simulink model "full_r2016b"  (R2019b)
settings: Solver=VariableStepAuto  StartTime=0.0  StopTime=10.0  RelTol=1e-3
libraries: aerolibgravity2 x2, aerolibconvert2 x1, vrlib x1
settings Model: Creator=decla  LastModifiedBy=decla
settings DebuggingCC: ArithmeticOperatorsInVariantConditions=warning
settings SFSimCC: CustomCodeUndefinedFunction=UseInterfaceOnly
settings CodeAppCC: StateflowObjectComments=on

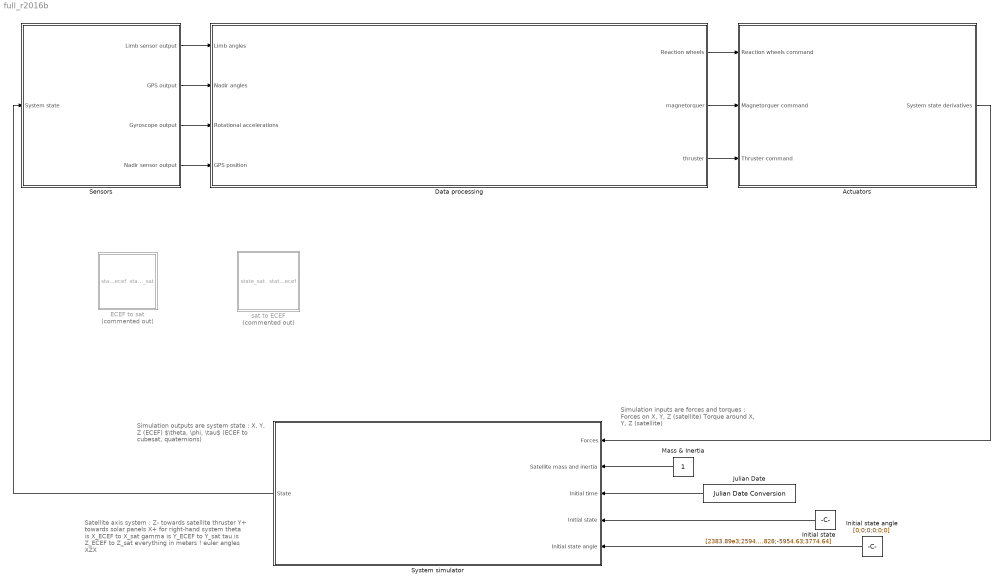
== system full_r2016b ==
  note: Simulation outputs are system state :
      | X, Y, Z (ECEF)
      | $\theta, \phi, \tau$ (ECEF to cubesat, quaternions)
  note: Simulation inputs are forces and torques :
      | Forces on X, Y, Z (satellite)
      | Torque around X, Y, Z (satellite)
  note: Satellite axis system :
      | Z- towards satellite thruster
      | Y+ towards solar panels
      | X+ for right-hand system
      | theta is X_ECEF to X_sat
      | gamma is Y_ECEF to Y_sat
      | tau is Z_ECEF to Z_sat
      | everything in meters !
      | euler angles XZX
  Actuators : Subsystem
  Data processing : Subsystem
  ECEF to sat : MATLAB Function  Commented=on  TreatAsAtomicUnit=on
  Initial state : Constant  Value=[2383.89e3;2594.67e3;5906.12e3;-2871.828;-5954.63;3774.64]
  Initial state angle : Constant  Value=[0;0;0;0;0;0]
  Julian Date : aerolibconvert2/Julian Date Conversion  year=2004  month=October  day=10  hour=12  min=21  sec=0  modflag=off  deltaT=None  errorflag=Error
      settings: SourceProductBaseCode=AE
  Mass & Inertia : Constant
  Sensors : Subsystem
  System simulator : Subsystem
  sat to ECEF : MATLAB Function  Commented=on  TreatAsAtomicUnit=on
  wires:
  Data processing/3(thruster) -> Actuators/3(Thruster command)
  Actuators/1(System state derivatives) -> System simulator/1(Forces)
  System simulator/1(State) -> Sensors/1(System state)
  Sensors/4(Nadir sensor output) -> Data processing/4(GPS position)
  Sensors/3(Gyroscope output) -> Data processing/3(Rotational accelerations)
  Sensors/2(GPS output) -> Data processing/2(Nadir angles)
  Sensors/1(Limb sensor output) -> Data processing/1(Limb angles)
  Data processing/2(magnetorquer) -> Actuators/2(Magnetorquer command)
  Data processing/1(Reaction wheels) -> Actuators/1(Reaction wheels command)
  Mass & Inertia/1 -> System simulator/2(Satellite mass and inertia)
  Julian Date/1 -> System simulator/3(Initial time)
  Initial state/1 -> System simulator/4(Initial state)
  Initial state angle/1 -> System simulator/5(Initial state angle)

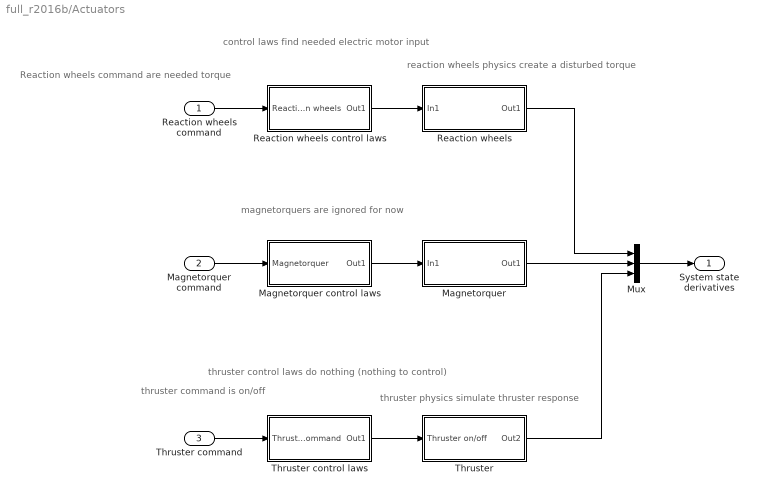
== system full_r2016b/Actuators ==
  note: magnetorquers are ignored for now
  note: thruster control laws do nothing (nothing to control)
  note: thruster physics simulate thruster response
  note: thruster command is on/off
  note: reaction wheels physics create a disturbed torque
  note: control laws find needed electric motor input
  note: Reaction wheels command are needed torque
  Reaction wheels command : Inport
  Magnetorquer command : Inport  Port=2
  Thruster command : Inport  Port=3
  Magnetorquer : Subsystem
  Magnetorquer control laws : Subsystem
  Mux : Mux  Inputs=3
  Reaction wheels : Subsystem
  Reaction wheels control laws : Subsystem
  Thruster : Subsystem
  Thruster control laws : Subsystem
  System state derivatives : Outport
  wires:
  Reaction wheels command/1 -> Reaction wheels control laws/1(Reaction wheels)
  Magnetorquer command/1 -> Magnetorquer control laws/1(Magnetorquer)
  Thruster command/1 -> Thruster control laws/1(Thruster command)
  Thruster control laws/1(Out1) -> Thruster/1(Thruster on/off)
  Magnetorquer control laws/1(Out1) -> Magnetorquer/1(In1)
  Reaction wheels control laws/1(Out1) -> Reaction wheels/1(In1)
  Thruster/1(Out2) -> Mux/3
  Magnetorquer/1(Out1) -> Mux/2
  Reaction wheels/1(Out1) -> Mux/1
  Mux/1 -> System state derivatives/1

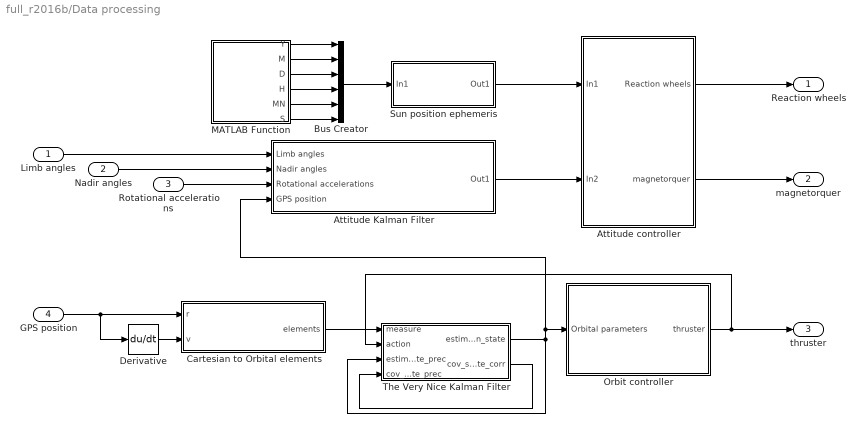
== system full_r2016b/Data processing ==
  Limb angles : Inport
  Nadir angles : Inport  Port=2
  Rotational accelerations : Inport  Port=3
  GPS position : Inport  Port=4
  Attitude Kalman Filter : Subsystem
  Attitude controller : Subsystem
  Bus Creator : BusCreator  Inputs=6
  Cartesian to Orbital elements : MATLAB Function  TreatAsAtomicUnit=on
  Derivative : Derivative
  MATLAB Function : MATLAB Function  TreatAsAtomicUnit=on
  Orbit controller : Subsystem
  Sun position ephemeris : Subsystem
  The Very Nice Kalman Filter : MATLAB Function  TreatAsAtomicUnit=on
  Reaction wheels : Outport
  magnetorquer : Outport  Port=2
  thruster : Outport  Port=3
  wires:
  Limb angles/1 -> Attitude Kalman Filter/1(Limb angles)
  Nadir angles/1 -> Attitude Kalman Filter/2(Nadir angles)
  Rotational accelerations/1 -> Attitude Kalman Filter/3(Rotational accelerations)
  Orbit controller/1(thruster) -> The Very Nice Kalman Filter/2(action), thruster/1
  Attitude controller/1(Reaction wheels) -> Reaction wheels/1
  Attitude controller/2(magnetorquer) -> magnetorquer/1
  MATLAB Function/1(Y) -> Bus Creator/1
  MATLAB Function/2(M) -> Bus Creator/2
  MATLAB Function/3(D) -> Bus Creator/3
  MATLAB Function/4(H) -> Bus Creator/4
  MATLAB Function/5(MN) -> Bus Creator/5
  MATLAB Function/6(S) -> Bus Creator/6
  Bus Creator/1 -> Sun position ephemeris/1(In1)
  Sun position ephemeris/1(Out1) -> Attitude controller/1(In1)
  Attitude Kalman Filter/1(Out1) -> Attitude controller/2(In2)
  Cartesian to Orbital elements/1(elements) -> The Very Nice Kalman Filter/1(measure)
  Derivative/1 -> Cartesian to Orbital elements/2(v)
  GPS position/1 -> Cartesian to Orbital elements/1(r), Derivative/1
  The Very Nice Kalman Filter/1(estimation_state) -> The Very Nice Kalman Filter/3(estimation_state_prec), Attitude Kalman Filter/4(GPS position), Orbit controller/1(Orbital parameters)
  The Very Nice Kalman Filter/2(cov_state_corr) -> The Very Nice Kalman Filter/4(cov_state_prec)

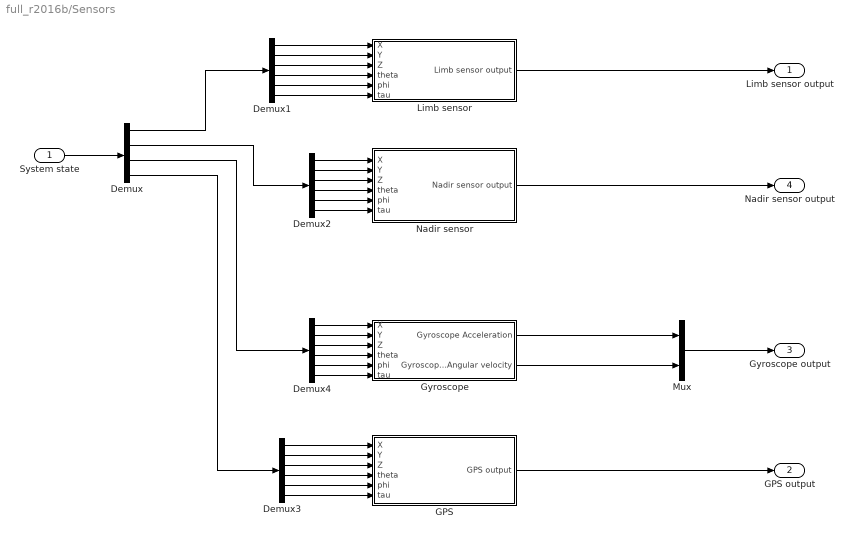
== system full_r2016b/Sensors ==
  System state : Inport
  Demux : Demux
  Demux{1..4} (4 alike) : Demux  Outputs=6
  GPS : Subsystem
  Gyroscope : Subsystem
  Limb sensor : Subsystem
  Mux : Mux  Inputs=2
  Nadir sensor : Subsystem
  Limb sensor output : Outport
  GPS output : Outport  Port=2
  Gyroscope output : Outport  Port=3
  Nadir sensor output : Outport  Port=4
  wires:
  Mux/1 -> Gyroscope output/1
  Demux1/1 -> Limb sensor/1(X)
  Demux1/4 -> Limb sensor/4(theta)
  Demux4/2 -> Gyroscope/2(Y)
  Demux1/5 -> Limb sensor/5(phi)
  Demux1/2 -> Limb sensor/2(Y)
  Demux3/1 -> GPS/1(X)
  Demux2/3 -> Nadir sensor/3(Z)
  Demux1/3 -> Limb sensor/3(Z)
  Demux4/1 -> Gyroscope/1(X)
  Demux3/3 -> GPS/3(Z)
  Demux2/6 -> Nadir sensor/6(tau)
  Limb sensor/1("Limb sensor output ") -> Limb sensor output/1
  GPS/1(GPS output) -> GPS output/1
  Demux4/3 -> Gyroscope/3(Z)
  Demux1/6 -> Limb sensor/6(tau)
  Demux3/4 -> GPS/4(theta)
  Demux2/1 -> Nadir sensor/1(X)
  Demux2/5 -> Nadir sensor/5(phi)
  Demux/1 -> Demux1/1
  Demux3/6 -> GPS/6(tau)
  Demux2/4 -> Nadir sensor/4(theta)
  Demux/3 -> Demux4/1
  Gyroscope/1(Gyroscope Acceleration) -> Mux/1
  Demux2/2 -> Nadir sensor/2(Y)
  Nadir sensor/1(Nadir sensor output) -> Nadir sensor output/1
  Gyroscope/2(Gyroscope Angular velocity) -> Mux/2
  Demux/4 -> Demux3/1
  Demux4/5 -> Gyroscope/5(phi)
  Demux4/4 -> Gyroscope/4(theta)
  Demux3/2 -> GPS/2(Y)
  Demux/2 -> Demux2/1
  Demux3/5 -> GPS/5(phi)
  Demux4/6 -> Gyroscope/6(tau)
  System state/1 -> Demux/1

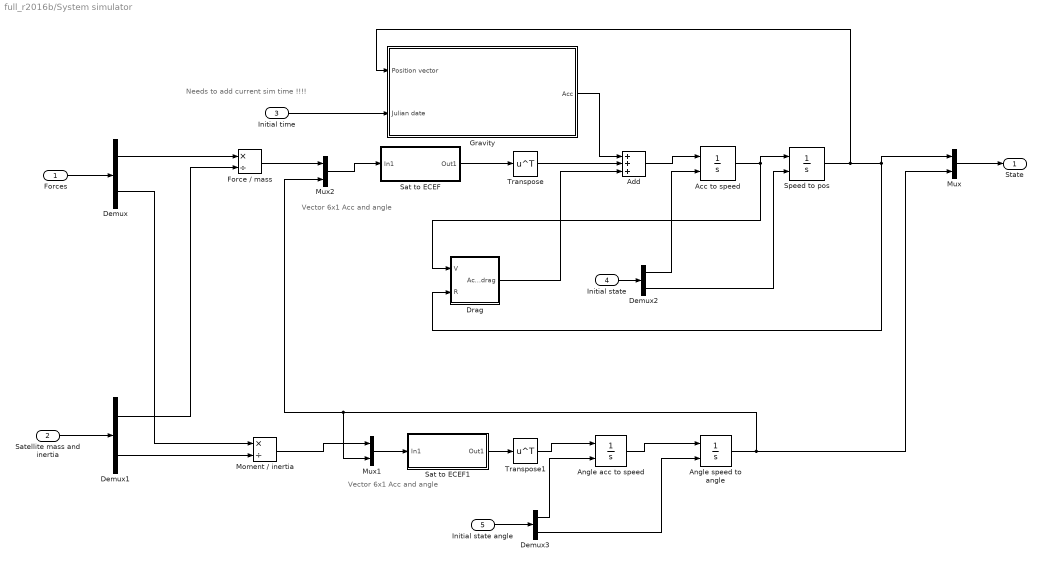
== system full_r2016b/System simulator ==
  note: Vector 6x1
      | Acc and angle
  note: Vector 6x1
      | Acc and angle
  note: Needs to add current sim time !!!!
  Forces : Inport
  Satellite mass and inertia : Inport  Port=2
  Initial time : Inport  Port=3
  Initial state : Inport  Port=4
  Initial state angle : Inport  Port=5
  Acc to speed : Integrator  InitialConditionSource=external  InitialCondition=[-2871.828;-5954.63;3774.64]
  Add : Sum  Inputs=+++
  Angle acc to speed : Integrator  InitialConditionSource=external
  Angle speed to angle : Integrator  InitialConditionSource=external
  Demux{,1..3} (4 alike) : Demux  Outputs=2
  Drag : Subsystem
  Force / mass : Product  Inputs=*/
  Gravity : Subsystem
  Moment / inertia : Product  Inputs=*/
  Mux : Mux  Inputs=2
  Mux1 : Mux  Inputs=2
  Mux2 : Mux  Inputs=2
  Sat to ECEF : Subsystem
  Sat to ECEF1 : Subsystem
  Speed to pos : Integrator  InitialConditionSource=external  InitialCondition=[2383.89e3;2594.67e3;5906.12e3]
  Transpose : Math  Operator=transpose  SaturateOnIntegerOverflow=on
  Transpose1 : Math  Operator=transpose  SaturateOnIntegerOverflow=on
  State : Outport
  wires:
  Add/1 -> Acc to speed/1
  Moment / inertia/1 -> Mux1/1
  Mux1/1 -> Sat to ECEF1/1(In1)
  Forces/1 -> Demux/1
  Force / mass/1 -> Mux2/1
  Mux2/1 -> Sat to ECEF/1(In1)
  Demux/1 -> Force / mass/1
  Demux1/2 -> Moment / inertia/2
  Mux/1 -> State/1
  Satellite mass and inertia/1 -> Demux1/1
  Angle speed to angle/1 -> Mux1/2, Mux2/2, Mux/2
  Sat to ECEF1/1(Out1) -> Transpose1/1
  Demux3/1 -> Angle acc to speed/2
  Initial state angle/1 -> Demux3/1
  Transpose/1 -> Add/2
  Demux3/2 -> Angle speed to angle/2
  Demux/2 -> Moment / inertia/1
  Transpose1/1 -> Angle acc to speed/1
  Demux2/2 -> Speed to pos/2
  Speed to pos/1 -> Mux/1, Drag/2(R), Gravity/1(Position vector)
  Gravity/1(Acc) -> Add/1
  Initial time/1 -> Gravity/2(Julian date)
  Angle acc to speed/1 -> Angle speed to angle/1
  Demux1/1 -> Force / mass/2
  Initial state/1 -> Demux2/1
  Acc to speed/1 -> Drag/1(V), Speed to pos/1
  Drag/1(Acc_drag) -> Add/3
  Demux2/1 -> Acc to speed/2
  Sat to ECEF/1(Out1) -> Transpose/1

== system full_r2016b/Actuators/Magnetorquer ==
  In1 : Inport
  Out1 : Outport
  wires:
  In1/1 -> Out1/1

== system full_r2016b/Actuators/Magnetorquer control laws ==
  Magnetorquer : Inport
  Out1 : Outport
  wires:
  Magnetorquer/1 -> Out1/1

== system full_r2016b/Actuators/Reaction wheels ==
  In1 : Inport
  Out1 : Outport
  wires:
  In1/1 -> Out1/1

== system full_r2016b/Actuators/Reaction wheels control laws ==
  Reaction wheels : Inport
  X wheel inertia : Constant
  Y wheel inertia1 : Constant
  Z wheel inertia1 : Constant
  Out1 : Outport
  wires:
  Reaction wheels/1 -> Out1/1

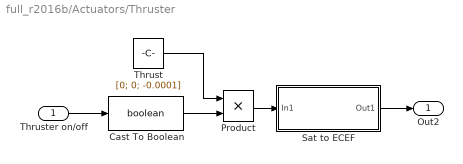
== system full_r2016b/Actuators/Thruster ==
  Thruster on/off : Inport
  Cast To Boolean : DataTypeConversion  OutDataTypeStr=boolean
  Product : Product
  Sat to ECEF : Subsystem
  Thrust : Constant  Value=[0; 0; -0.0001]
  Out2 : Outport
  wires:
  Product/1 -> Sat to ECEF/1(In1)
  Thrust/1 -> Product/1
  Thruster on/off/1 -> Cast To Boolean/1
  Sat to ECEF/1(Out1) -> Out2/1
  Cast To Boolean/1 -> Product/2

== system full_r2016b/Actuators/Thruster control laws ==
  Thruster command : Inport
  Out1 : Outport
  wires:
  Thruster command/1 -> Out1/1

== system full_r2016b/Data processing/Attitude Kalman Filter ==
  Limb angles : Inport
  Nadir angles : Inport  Port=2
  Rotational accelerations : Inport  Port=3
  GPS position : Inport  Port=4
  Out1 : Outport
  wires:
  Limb angles/1 -> Out1/1

== system full_r2016b/Data processing/Attitude controller ==
  In1 : Inport
  In2 : Inport  Port=2
  Command : Subsystem
  Control : Subsystem
  Reaction wheels : Outport
  magnetorquer : Outport  Port=2
  wires:
  In2/1 -> Control/3(In3)
  In1/1 -> Control/2(In2)
  Control/2(magnetorquer) -> magnetorquer/1
  Control/1(Reaction wheels) -> Reaction wheels/1
  Command/1(Out1) -> Control/1(In1)

== system full_r2016b/Data processing/Orbit controller ==
  Orbital parameters : Inport
  Command : Subsystem
  Control : Subsystem
  thruster : Outport
  wires:
  Command/1(Out1) -> Control/2(In1)
  Orbital parameters/1 -> Control/1(Orbital parameters)
  Control/1(Out1) -> thruster/1

== system full_r2016b/Data processing/Sun position ephemeris ==
  In1 : Inport
  Out1 : Outport
  wires:
  In1/1 -> Out1/1

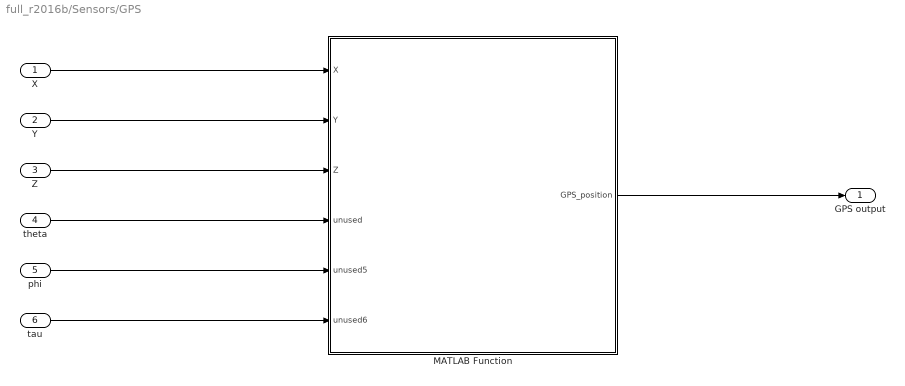
== system full_r2016b/Sensors/GPS ==
  X : Inport
  Y : Inport  Port=2
  Z : Inport  Port=3
  theta : Inport  Port=4
  phi : Inport  Port=5
  tau : Inport  Port=6
  MATLAB Function : MATLAB Function  TreatAsAtomicUnit=on
  GPS output : Outport
  wires:
  MATLAB Function/1(GPS_position) -> GPS output/1
  X/1 -> MATLAB Function/1(X)
  Y/1 -> MATLAB Function/2(Y)
  Z/1 -> MATLAB Function/3(Z)
  theta/1 -> MATLAB Function/4(unused)
  phi/1 -> MATLAB Function/5(unused5)
  tau/1 -> MATLAB Function/6(unused6)

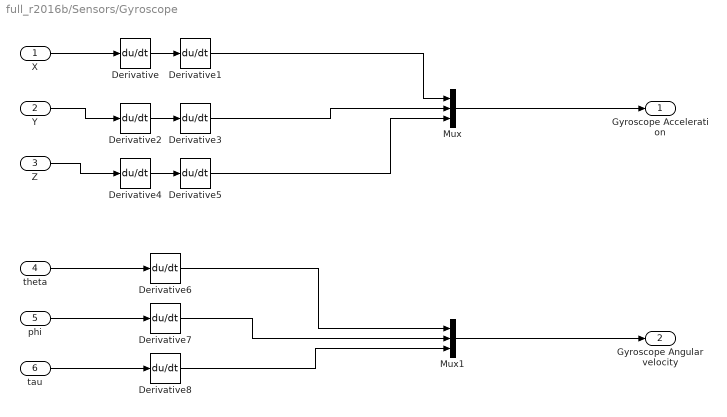
== system full_r2016b/Sensors/Gyroscope ==
  X : Inport
  Y : Inport  Port=2
  Z : Inport  Port=3
  theta : Inport  Port=4
  phi : Inport  Port=5
  tau : Inport  Port=6
  Derivative{,1..8} (9 alike) : Derivative
  Mux : Mux  Inputs=3
  Mux1 : Mux  Inputs=3
  Gyroscope Acceleration : Outport
  Gyroscope Angular velocity : Outport  Port=2
  wires:
  Derivative/1 -> Derivative1/1
  Derivative1/1 -> Mux/1
  X/1 -> Derivative/1
  Derivative2/1 -> Derivative3/1
  Derivative3/1 -> Mux/2
  Derivative4/1 -> Derivative5/1
  Derivative5/1 -> Mux/3
  Mux/1 -> Gyroscope Acceleration/1
  Z/1 -> Derivative4/1
  Y/1 -> Derivative2/1
  theta/1 -> Derivative6/1
  phi/1 -> Derivative7/1
  tau/1 -> Derivative8/1
  Derivative6/1 -> Mux1/1
  Derivative7/1 -> Mux1/2
  Derivative8/1 -> Mux1/3
  Mux1/1 -> Gyroscope Angular velocity/1

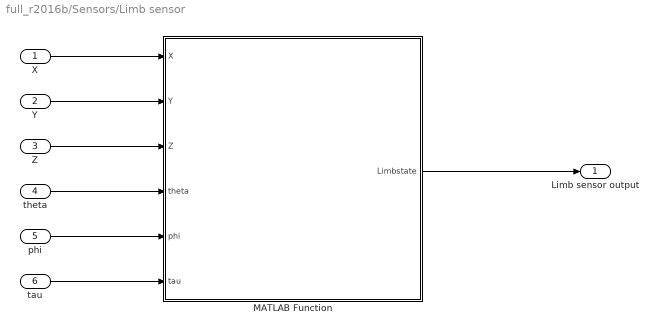
== system full_r2016b/Sensors/Limb sensor ==
  X : Inport
  Y : Inport  Port=2
  Z : Inport  Port=3
  theta : Inport  Port=4
  phi : Inport  Port=5
  tau : Inport  Port=6
  MATLAB Function : MATLAB Function  TreatAsAtomicUnit=on
  "Limb sensor output " : Outport
  wires:
  X/1 -> MATLAB Function/1(X)
  MATLAB Function/1(Limbstate) -> "Limb sensor output "/1
  tau/1 -> MATLAB Function/6(tau)
  phi/1 -> MATLAB Function/5(phi)
  theta/1 -> MATLAB Function/4(theta)
  Z/1 -> MATLAB Function/3(Z)
  Y/1 -> MATLAB Function/2(Y)

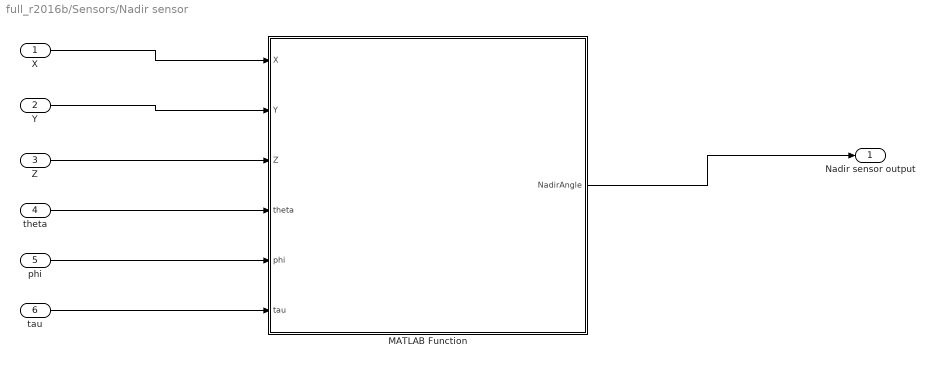
== system full_r2016b/Sensors/Nadir sensor ==
  X : Inport
  Y : Inport  Port=2
  Z : Inport  Port=3
  theta : Inport  Port=4
  phi : Inport  Port=5
  tau : Inport  Port=6
  MATLAB Function : MATLAB Function  TreatAsAtomicUnit=on
  Nadir sensor output : Outport
  wires:
  MATLAB Function/1(NadirAngle) -> Nadir sensor output/1
  X/1 -> MATLAB Function/1(X)
  Y/1 -> MATLAB Function/2(Y)
  Z/1 -> MATLAB Function/3(Z)
  theta/1 -> MATLAB Function/4(theta)
  phi/1 -> MATLAB Function/5(phi)
  tau/1 -> MATLAB Function/6(tau)

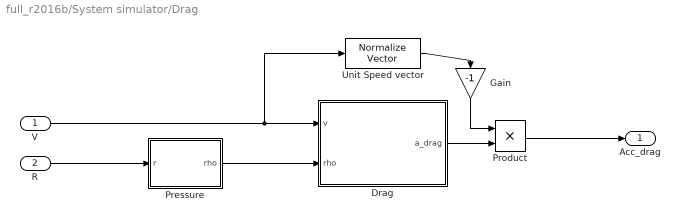
== system full_r2016b/System simulator/Drag ==
  V : Inport
  R : Inport  Port=2
  Drag : MATLAB Function  TreatAsAtomicUnit=on
  Gain : Gain  Gain=-1
  Pressure : MATLAB Function  TreatAsAtomicUnit=on
  Product : Product
  Unit Speed vector : vrlib/Utilities/Normalize Vector  maxzero=0
  Acc_drag : Outport
  wires:
  Pressure/1(rho) -> Drag/2(rho)
  V/1 -> Unit Speed vector/1, Drag/1(v)
  R/1 -> Pressure/1(r)
  Unit Speed vector/1 -> Gain/1
  Product/1 -> Acc_drag/1
  Drag/1(a_drag) -> Product/2
  Gain/1 -> Product/1

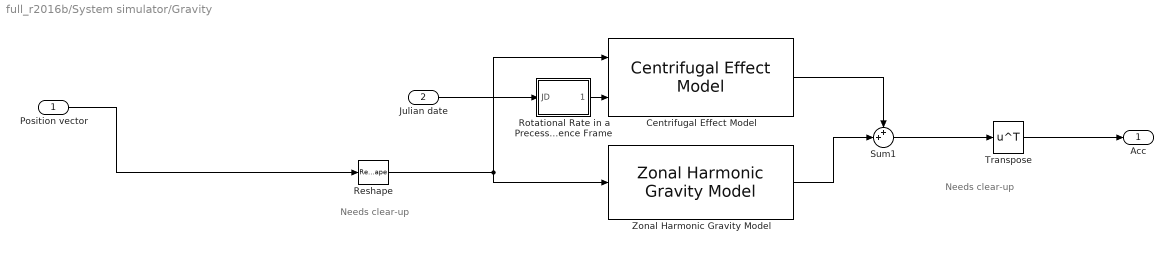
== system full_r2016b/System simulator/Gravity ==
  note: Needs clear-up
  note: Needs clear-up
  Position vector : Inport
  Julian date : Inport  Port=2
  Centrifugal Effect Model : aerolibgravity2/Centrifugal Effect Model  ptype=Custom  omega=7.2921150e-005  rate_loc=on
      settings: SourceProductBaseCode=AE
  Reshape : Reshape  OutputDimensionality=Row vector (2-D)
  Rotational Rate in a Precessing Reference Frame : Subsystem
  Sum1 : Sum  Inputs=++|
  Transpose : Math  Operator=transpose  SignedPower=on  SaturateOnIntegerOverflow=on
  Zonal Harmonic Gravity Model : aerolibgravity2/Zonal Harmonic Gravity Model  units=Metric (MKS)  degree=4  action=Warning  ptype=Earth  R=6378136.3  GM=398600441500000  jvalue=[1.0826269e-03 -2.5323000e-06 -1.6204000e-06]
      settings: SourceProductBaseCode=AE
  Acc : Outport
  wires:
  Reshape/1 -> Centrifugal Effect Model/1, Zonal Harmonic Gravity Model/1
  Rotational Rate in a Precessing Reference Frame/1(omega) -> Centrifugal Effect Model/2
  Position vector/1 -> Reshape/1
  Julian date/1 -> Rotational Rate in a Precessing Reference Frame/1(JD)
  Zonal Harmonic Gravity Model/1 -> Sum1/2
  Centrifugal Effect Model/1 -> Sum1/1
  Sum1/1 -> Transpose/1
  Transpose/1 -> Acc/1

== system full_r2016b/System simulator/Sat to ECEF ==
  In1 : Inport
  SAT TO ECEF : MATLAB Function  TreatAsAtomicUnit=on
  Out1 : Outport
  wires:
  In1/1 -> SAT TO ECEF/1(state_sat)
  SAT TO ECEF/1(state_ecef) -> Out1/1

== system full_r2016b/System simulator/Sat to ECEF1 ==
  In1 : Inport
  SAT TO ECEF : MATLAB Function  TreatAsAtomicUnit=on
  Out1 : Outport
  wires:
  In1/1 -> SAT TO ECEF/1(state_sat)
  SAT TO ECEF/1(state_ecef) -> Out1/1

== system full_r2016b/Actuators/Thruster/Sat to ECEF ==
  In1 : Inport
  Out1 : Outport
  wires:
  In1/1 -> Out1/1

== system full_r2016b/Data processing/Attitude controller/Command ==
  In1 : Inport
  Out1 : Outport
  wires:
  In1/1 -> Out1/1

== system full_r2016b/Data processing/Attitude controller/Control ==
  In1 : Inport
  In2 : Inport  Port=2
  In3 : Inport  Port=3
  Reaction wheels : Outport
  magnetorquer : Outport  Port=2
  wires:
  In1/1 -> Reaction wheels/1

== system full_r2016b/Data processing/Orbit controller/Command ==
  In1 : Inport
  Constant : Constant
  Out1 : Outport
  wires:
  In1/1 -> Out1/1

== system full_r2016b/Data processing/Orbit controller/Control ==
  Orbital parameters : Inport
  In1 : Inport  Port=2
  Out1 : Outport
  wires:
  Orbital parameters/1 -> Out1/1

== system full_r2016b/System simulator/Gravity/Rotational Rate in a Precessing Reference Frame ==
  JD : Inport
  Bias : Bias  Bias=-2451545
  Bias1 : Bias  Bias=7.086e-12
  Bias2 : Bias  Bias=7.2921151467e-5
  Gain : Gain  Gain=4.3e-15/36525
  omega : Outport
  wires:
  JD/1 -> Bias/1
  Bias/1 -> Gain/1
  Gain/1 -> Bias1/1
  Bias1/1 -> Bias2/1
  Bias2/1 -> omega/1

== matlab function full_r2016b/ECEF to sat ==
  data: state_ecef input; state_sat output
function state_sat = fcn(state_ecef)

    x = state(0)
    y = state(1)
    z = state(2)
    theta = state(3)
    phi = state(4)
    tau = state(5)

    % from https://en.wikipedia.org/wiki/Euler_angles
    c1 = cos(theta)
    c2 = cos(phi)
    c3 = cos(tau)
    s1 = sin(theta)
    s2 = sin(phi)
    s3 = sin(tau)
    XZX = [
       c2, -c3*c2, s2*s3;
       c1*s2, c1*c2*c3-s1*s3, -c3*s1-c1*c2*s3;
       s1*s2, c1*s3+c2*c3*s1, c1*c3-c2*s1*s3
    ];
    
    state_sat =[x;y;z]*XZX;

== matlab function full_r2016b/Data processing/MATLAB Function ==
  data: Y output; M output; D output; H output; MN output; S output
% https://www.mathworks.com/matlabcentral/answers/30479-how-to-get-system-date-and-time-into-simulink
function [Y, M, D, H, MN, S] = sysClock()
   coder.extrinsic('clock');
   Y = 0;
   M = 0;
   D = 0;
   H = 0;
   MN = 0;
   S = 0;
   [Y, M, D, H, MN, S] = clock;
end

== matlab function full_r2016b/System simulator/Drag/Drag ==
  data: v input; a_drag output; rho input
function a_drag = fcn(v, rho)
area = 100e-4;
mass = 3;
V = norm(v);
Cd = 1.05;

a_drag = -0.5*Cd*(area/mass)*rho*V^2;

== matlab function full_r2016b/System simulator/Drag/Pressure ==
  data: r input; rho output
function rho = fcn(r)
alt = norm(r);
A = 1.140564e-10;
B = -2.130756e-7;
C = 1.570562e-4;
D = -0.07029296;
E = -12.89844;

rho = exp(A*alt^4 + B*alt^3 + C*alt^2 + D*alt + E);

== matlab function full_r2016b/Sensors/GPS/MATLAB Function ==
  data: X input; GPS_position output; Y input; Z input; unused input; unused5 input; unused6 input
function GPS_position    = GPS_function(X, Y, Z, ~, ~, ~)


noise_pos = 0 + (10-0) .* rand(1,1); % bruit pour la position X
GPS_position_x = X + noise_pos;
noise_pos = 0 + (10-0) .* rand(1,1); % bruit pour la position Y
GPS_position_y = Y + noise_pos;
noise_pos = 0 + (10-0) .* rand(1,1); % bruit pour la position Z
GPS_position_z = Z + noise_pos;

GPS_position = [GPS_position_x; GPS_position_y; GPS_position_z];
end

== matlab function full_r2016b/Sensors/Limb sensor/MATLAB Function ==
  data: X input; Limbstate output; Y input; Z input; theta input; phi input; tau input
function Limbstate  = Limb_function(X, Y, Z, theta, phi, tau)
% Take as input the postition X,Y,Z and the attitude Theta (rotX), phi
% (rotY), tau (rotZ).
% Return the limb state in ECEF ref 

noise = 0 + (0.25-0) .* rand(1,1);
LimbAngle = acrtan(6371000/ sqrt(X^2 + Y^2 + Z^2)) + noise; % Tan(angle) = opposite * Adj

tau2limb = tau - limbAngle  % angle between tau and limb  




c1 = cos(theta)
c2 = cos(phi)
c3 = cos(tau2limb)
s1 = sin(theta)
s2 = sin(phi)
s3 = sin(tau2limb)
XZX = [
c2, -c3*c2, s2*s3;
c1*s2, c1*c2*c3-s1*s3, -c3*s1-c1*c2*s3;
s1*s2, c1*s3+c2*c3*s1, c1*c3-c2*s1*s3
];

Limbstate =[X;Y;Z]*(XZX');

end

== matlab function full_r2016b/Sensors/Nadir sensor/MATLAB Function ==
  data: X input; NadirAngle output; Y input; Z input; theta input; phi input; tau input
function NadirAngle   = Nadir_function(X, Y, Z, theta, phi, tau)
% En faisant l'hypothèse que SystemStates = ([rotX rotY rotZ],[X Y Z])
noise = 0 + (0.25-0) .* rand(1,1);
NadirAngle_x = -X + noise;
noise = 0 + (0.25-0) .* rand(1,1);
NadirAngle_y = -Y + noise;
noise = 0 + (0.25-0) .* rand(1,1);
NadirAngle_z = -Z + noise;


vector = -1 .* [NadirAngle_x, NadirAngle_y, NadirAngle_z];

unit_vector = vector / (sqrt(NadirAngle_x^2 + NadirAngle_y^2 + NadirAngle_z^2)


% from https://en.wikipedia.org/wiki/Euler_angles
c1 = cos(theta)
c2 = cos(phi)
c3 = cos(tau)
s1 = sin(theta)
s2 = sin(phi)
s3 = sin(tau)
XZX = [
c2, -c3*c2, s2*s3;
c1*s2, c1*c2*c3-s1*s3, -c3*s1-c1*c2*s3;
s1*s2, c1*s3+c2*c3*s1, c1*c3-c2*s1*s3
];

state_sat =unit_vector .* XZX;
end

== matlab function full_r2016b/sat to ECEF ==
  data: state_sat input; state_ecef output
function state_ecef = fcn(state_sat)

    x = state(0)
    y = state(1)
    z = state(2)
    theta = state(3)
    phi = state(4)
    tau = state(5)

    % from https://en.wikipedia.org/wiki/Euler_angles
    c1 = cos(theta)
    c2 = cos(phi)
    c3 = cos(tau)
    s1 = sin(theta)
    s2 = sin(phi)
    s3 = sin(tau)
    XZX = [
       c2, -c3*c2, s2*s3;
       c1*s2, c1*c2*c3-s1*s3, -c3*s1-c1*c2*s3;
       s1*s2, c1*s3+c2*c3*s1, c1*c3-c2*s1*s3
    ];
    
    state_ecef =[x;y;z]*(XZX');

== matlab function full_r2016b/Data processing/Cartesian to Orbital elements ==
  data: r input; elements output; v input
function elements = to_orbital(r,v)
    % r is x;y;z
    % v is dx;dy;dz
    
    mu = 398600;h = cross(r,v);
    nR = norm(r); nV = norm(v);
    a = (2 /nR - nV^2 / mu)^(-1);
    e = 1 / mu * (cross(v,h) - mu * r ./nR);
    nE = norm(e);
    i = acos(h(3) /norm(h));
    k = [0; 0; 1];
    n = cross(k,h);
    
    if (n(2) < 0)
        Omega = 2 * pi - arccos(n(1)/norm(n));
    else
        Omega = acos(n(1)/norm(n));
    end
    if (e(3) < 0)
        omega = 2 * pi - acos(dot(n, e)/(norm(n)* norm(e)));
    else
        omega = acos(dot(n, e)/(norm(n)* norm(e)));
    end
    
    % theta0 is true anomaly
    if (dot(r, v) < 0)
        theta0 = 2 * pi - acos(dot(e, r)/(norm(e)* norm(r0)));
    else
        theta0 = acos(dot(e, r)/(norm(e)* norm(r)));
    end
    
    elements = [a, nE, i, Omega, omega, theta0];

== matlab function full_r2016b/Data processing/The Very Nice Kalman Filter ==
  data: measure input; estimation_state output; action input; estimation_state_prec input; cov_state_prec input; cov_state_corr output
function [estimation_state, cov_state_corr]= gps_kalman(measure, action, estimation_state_prec, cov_state_prec) 

    % measure = [a, e, i, Omega, omega, theta0] 
    % state = [a, e, i, Omega, omega, theta0] 

    R = % measure noise covariance
    Q = % state noise covariance
    
    % to find : linearize equations around current state
    
    F = % df/dx
    G = % df/du
    H = % df/d noise
    C = % dh/dx
    D = % dh/du
    L = % dh/d noise
    
    % mu = 398600
    theta_dot = sqrt(mu*a*(1-(e^2)))/(norm((a*(1-(e^2)))/(1+(e*cos(theta0_prec))))^2) % space cheat sheet from Valispace
    state_est = [a_prec; e_prec; i_prec; Omega_prec; omega_prec; theta_prec + (theta_dot*gps_sample_time)];
    measure_est = [1; 1; 1; 1; 1; 1];

    
    cov_state = F*cov_state_prec*F' + H*Q*H'
    cov_output = C*cov_state*C' + L*R*L'
    
    K = cov_state*C'*cov_output 
    estimation_state = state_est + K*(measure - measure_est)
    cov_state_corr = cov_state - K*C*cov_state

== matlab function full_r2016b/System simulator/Sat to ECEF/SAT TO ECEF ==
  data: state_sat input; state_ecef output
function state_ecef = fcn(state_sat)

x = state_sat(0);
y = state_sat(1);
z = state_sat(2);
theta = state_sat(3);
phi = state_sat(4);
tau = state_sat(5);

% from https://en.wikipedia.org/wiki/Euler_angles
c1 = cos(theta);
c2 = cos(phi);
c3 = cos(tau);
s1 = sin(theta);
s2 = sin(phi);
s3 = sin(tau);
XZX = [
c2, -c3*c2, s2*s3;
c1*s2, c1*c2*c3-s1*s3, -c3*s1-c1*c2*s3;
s1*s2, c1*s3+c2*c3*s1, c1*c3-c2*s1*s3
];

state_ecef =[x;y;z]*(XZX');

== matlab function full_r2016b/System simulator/Sat to ECEF1/SAT TO ECEF ==
  data: state_sat input; state_ecef output
function state_ecef = fcn(state_sat)

x = state_sat(0);
y = state_sat(1);
z = state_sat(2);
theta = state_sat(3);
phi = state_sat(4);
tau = state_sat(5);

% from https://en.wikipedia.org/wiki/Euler_angles
c1 = cos(theta);
c2 = cos(phi);
c3 = cos(tau);
s1 = sin(theta);
s2 = sin(phi);
s3 = sin(tau);
XZX = [
c2, -c3*c2, s2*s3;
c1*s2, c1*c2*c3-s1*s3, -c3*s1-c1*c2*s3;
s1*s2, c1*s3+c2*c3*s1, c1*c3-c2*s1*s3
];

state_ecef =[x;y;z]*(XZX');
